simulink model "Controlador_ScripDiscreto"  (R2013b)
settings: Solver=ode45  StartTime=0.0  StopTime=10.0  RelTol=1e-3
values from neighbouring files (symbols this model uses):
  A = [-1.01887   0.90506   -0.00215 ... (first row only)    [Robustez.m]
  B = [0  0  20.2]'    [Robustez.m]
  C = [57.2958      0    0 ... (first row only)    [Robustez.m]
  D = [0 0]'    [Robustez.m]
undefined symbols (not defined in the file or in its folder): dt
settings Model: Creator=Eduardo  LastModifiedBy=Eduardo

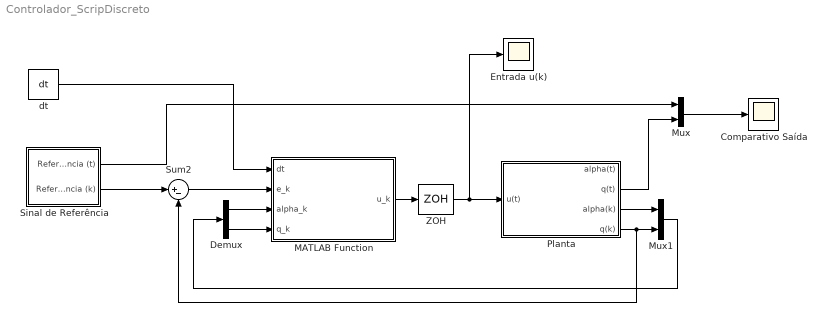
== system Controlador_ScripDiscreto ==
  Comparativo Saída : Scope
  Demux : Demux  Outputs=2
  Entrada u(k) : Scope
  MATLAB Function : MATLAB Function  TreatAsAtomicUnit=on
  Mux : Mux  Inputs=2
  Mux1 : Mux  Inputs=2
  "Planta " : Subsystem
  Sinal de Referência : Subsystem
  Sum2 : Sum  Inputs=|+-
  "ZOH  " : ZeroOrderHold  SampleTime=dt
  dt : Constant  Value=dt
  wires:
  Mux/1 -> Comparativo Saída/1
  Sinal de Referência/2(Referência (k)) -> Sum2/1
  "Planta "/3(alpha(k)) -> Mux1/1
  "Planta "/4(q(k)) -> Sum2/2, Mux1/2
  Demux/1 -> MATLAB Function/3(alpha_k)
  Demux/2 -> MATLAB Function/4(q_k)
  Mux1/1 -> Demux/1
  Sum2/1 -> MATLAB Function/2(e_k)
  dt/1 -> MATLAB Function/1(dt)
  MATLAB Function/1(u_k) -> "ZOH  "/1
  Sinal de Referência/1(Referência (t)) -> Mux/1
  "Planta "/2(q(t)) -> Mux/2
  "ZOH  "/1 -> Entrada u(k)/1, "Planta "/1(u(t))

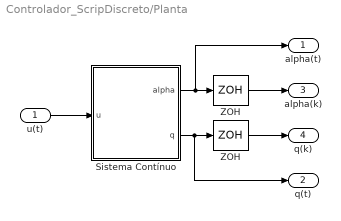
== system Controlador_ScripDiscreto/Planta  ==
  u(t) : Inport
  "Sistema Contínuo " : Subsystem
  ZOH : ZeroOrderHold  SampleTime=dt
  "ZOH  " : ZeroOrderHold  SampleTime=dt
  alpha(t) : Outport
  q(t) : Outport  Port=2
  alpha(k) : Outport  Port=3
  q(k) : Outport  Port=4
  wires:
  "ZOH  "/1 -> q(k)/1
  ZOH/1 -> alpha(k)/1
  u(t)/1 -> "Sistema Contínuo "/1(u)
  "Sistema Contínuo "/2(q) -> "ZOH  "/1, q(t)/1
  "Sistema Contínuo "/1(alpha) -> alpha(t)/1, ZOH/1

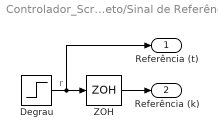
== system Controlador_ScripDiscreto/Sinal de Referência ==
  note: r
  Degrau : Step  Time=0  SampleTime=0
  "ZOH " : ZeroOrderHold  SampleTime=dt
  Referência (t) : Outport
  Referência (k) : Outport  Port=2
  wires:
  Degrau/1 -> Referência (t)/1, "ZOH "/1
  "ZOH "/1 -> Referência (k)/1

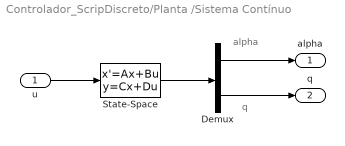
== system Controlador_ScripDiscreto/Planta /Sistema Contínuo  ==
  note: alpha
  note: q
  u : Inport
  Demux : Demux  Outputs=2
  State-Space : StateSpace  A=A  B=B  C=C  D=D  X0=0
  alpha : Outport
  q : Outport  Port=2
  wires:
  State-Space/1 -> Demux/1
  u/1 -> State-Space/1
  Demux/2 -> q/1
  Demux/1 -> alpha/1

== matlab function Controlador_ScripDiscreto/MATLAB Function ==
  data: dt input; e_k input; u_k output; alpha_k input; q_k input
function u_k = fcn(dt, e_k, alpha_k, q_k)

persistent e_k1
persistent alpha_k1
persistent q_k1

persistent v1_k1
persistent v2_k1


% Inicialização das constantes do controlador.
% --------------------------------------------
if (isempty(e_k1))
    e_k1 = 0;
end
if (isempty(alpha_k1))
    alpha_k1 = 0;
end
if (isempty(q_k1))
    q_k1 = 0;
end

if (isempty(v1_k1))
    v1_k1 = 0;
end
if (isempty(v2_k1))
    v2_k1 = 0;
end


% Obtidos na página 594 do livro do Lewis.
% ----------------------------------------
Ki = 1.361;
Ka = -0.0807;
Kq = -0.475;

% Ganhos já discretizados.
% ------------------------
k1 = Ki*dt/2;
PI = (1-10*dt/2)/(1+10*dt/2);
k2 = 10*Ka*dt/(10*dt+2);
k3 = Kq;

% Parâmetros do sistema.
v1_k = v1_k1 + k1*(e_k + e_k1);
v2_k = PI*v2_k1 + k2*(alpha_k + alpha_k1);
v3_k = k3*q_k;



% Atualização dos valores persistentes.
% -------------------------------------
e_k1     = e_k;
alpha_k1 = alpha_k;
q_k1     = q_k;
v1_k1    = v1_k;
v2_k1    = v2_k;

% Valor do controle a ser aplicado à planta.
% ------------------------------------------
u_k = -(v1_k + v2_k + v3_k);
